simulink model "Battery_Equivalent_circuit"  (R2023b)
settings: Solver=ode23t  StartTime=0.0  StopTime=3600  MaxStep=1  RelTol=1e-3
libraries: fl_lib x11, nesl_utility x5
settings Model: Creator=prade  LastModifiedBy=prade
settings DataIOCC: SignalLoggingName=Battery_Equivalent_circuit
settings SimscapeCC: SimscapeLogType=all  SimscapeLogSimulationStatistics=on  SimscapeLogName=Battery_Equivalent_circuit

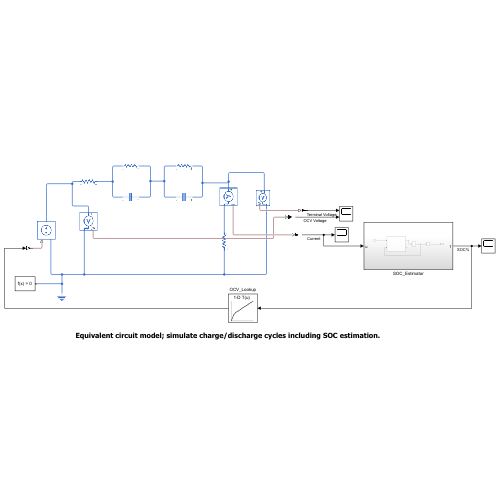
[thumbnail: Simulink's stored preview of the top-level diagram]
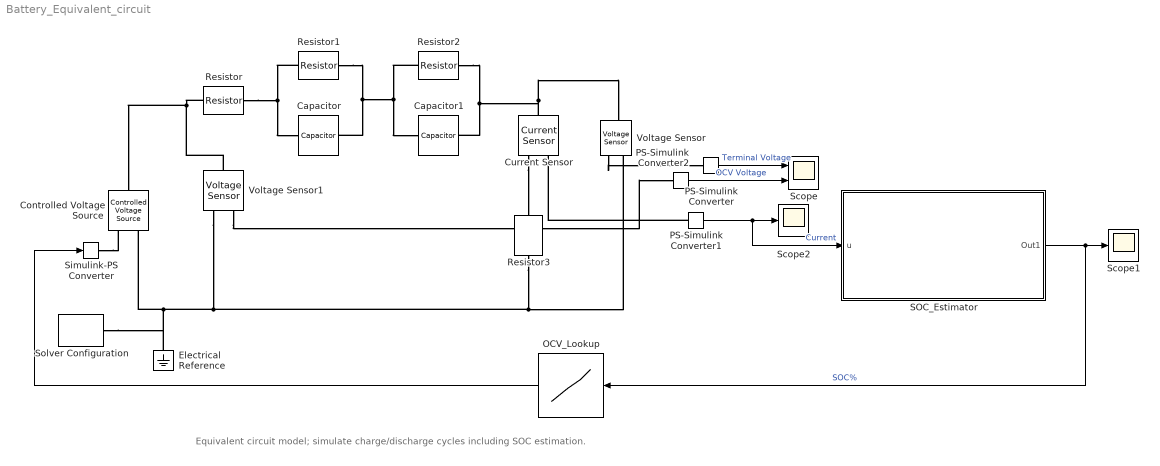
== system Battery_Equivalent_circuit ==
  note: Equivalent circuit model; simulate charge/discharge cycles including SOC estimation.
  Capacitor : fl_lib/Electrical/Electrical Elements/Capacitor  c=1000 F  r=1e-6 Ohm  g=0 1/Ohm  i_specify=off  i_priority=None  i=0 A  i_nominal_specify=off  i_nominal_unit=A  i_nominal_value=1  v_specify=off  v_priority=None  v=0 V  v_nominal_specify=off  v_nominal_unit=V  v_nominal_value=1  vc_specify=off  vc_priority=High  vc=0 V  vc_nominal_specify=off  vc_nominal_unit=V  vc_nominal_value=1
  Capacitor1 : fl_lib/Electrical/Electrical Elements/Capacitor  c=10000 F  r=1e-6 Ohm  g=0 1/Ohm  i_specify=off  i_priority=None  i=0 A  i_nominal_specify=off  i_nominal_unit=A  i_nominal_value=1  v_specify=off  v_priority=None  v=0 V  v_nominal_specify=off  v_nominal_unit=V  v_nominal_value=1  vc_specify=off  vc_priority=High  vc=0 V  vc_nominal_specify=off  vc_nominal_unit=V  vc_nominal_value=1
  Controlled Voltage Source : fl_lib/Electrical/Electrical Sources/Controlled Voltage Source
  Current Sensor : fl_lib/Electrical/Electrical Sensors/Current Sensor
  Electrical Reference : fl_lib/Electrical/Electrical Elements/Electrical Reference
  OCV_Lookup : Lookup_n-D  NumberOfTableDimensions=1  BreakpointsForDimension1=[0 10 20 30 40 50 60 70 80 90 100]  Table=[2.8 3.2 3.4 3.5 3.6 3.7 3.8 3.9 4.0 4.1 4.2]  InternalRulePriority=Speed  RndMeth=Simplest
  PS-Simulink Converter : nesl_utility/PS-Simulink Converter  PhysicalDomain=network_engine_domain  SubClassName=ps_output  LeftPortType=input  RightPortType=output  PseudoPeriodic=off  Frequencies=[]  VectorFormat=inherit  Unit=inherit  AffineConversion=off
  PS-Simulink Converter1 : nesl_utility/PS-Simulink Converter  PhysicalDomain=network_engine_domain  SubClassName=ps_output  LeftPortType=input  RightPortType=output  PseudoPeriodic=off  Frequencies=[]  VectorFormat=inherit  Unit=inherit  AffineConversion=off
  PS-Simulink Converter2 : nesl_utility/PS-Simulink Converter  PhysicalDomain=network_engine_domain  SubClassName=ps_output  LeftPortType=input  RightPortType=output  PseudoPeriodic=off  Frequencies=[]  VectorFormat=inherit  Unit=inherit  AffineConversion=off
  Resistor : fl_lib/Electrical/Electrical Elements/Resistor  R=0.05 Ohm  i_specify=off  i_priority=None  i=0 A  i_nominal_specify=off  i_nominal_unit=A  i_nominal_value=1  v_specify=off  v_priority=None  v=0 V  v_nominal_specify=off  v_nominal_unit=V  v_nominal_value=1
  Resistor1 : fl_lib/Electrical/Electrical Elements/Resistor  R=0.02 Ohm  i_specify=off  i_priority=None  i=0 A  i_nominal_specify=off  i_nominal_unit=A  i_nominal_value=1  v_specify=off  v_priority=None  v=0 V  v_nominal_specify=off  v_nominal_unit=V  v_nominal_value=1
  Resistor2 : fl_lib/Electrical/Electrical Elements/Resistor  R=0.01 Ohm  i_specify=off  i_priority=None  i=0 A  i_nominal_specify=off  i_nominal_unit=A  i_nominal_value=1  v_specify=off  v_priority=None  v=0 V  v_nominal_specify=off  v_nominal_unit=V  v_nominal_value=1
  Resistor3 : fl_lib/Electrical/Electrical Elements/Resistor  R=3.7 Ohm  i_specify=off  i_priority=None  i=0 A  i_nominal_specify=off  i_nominal_unit=A  i_nominal_value=1  v_specify=off  v_priority=None  v=0 V  v_nominal_specify=off  v_nominal_unit=V  v_nominal_value=1
  SOC_Estimator : Subsystem
  Scope : Scope  NumInputPorts=2
  Scope1 : Scope
  Scope2 : Scope
  Simulink-PS Converter : nesl_utility/Simulink-PS Converter  PhysicalDomain=network_engine_domain  SubClassName=ps_input  LeftPortType=input  RightPortType=output  PseudoPeriodic=off  Frequencies=[]  NoiseDistribution=none  NoiseParameters=[]  Unit=1  AffineConversion=off  FilteringAndDerivatives=provide  SimscapeFilterOrder=1  InputFilterTimeConstant=0.001  UdotUserProvided=0
  Solver Configuration : nesl_utility/Solver Configuration  PhysicalDomain=network_engine_domain  SubClassName=solver  LeftPortType=input  RightPortType=generic  Tones=[]  Harmonics=[]  SimulateNoise=off  Profile=off  UseLocalSampling=off  EnableSwitchedLinearOptims=on  FrequencyDomain=off  UseCCode=off  RelTol=0.001  AbsTol=0.001  MinStep=1e-09  ToWorkspace=off  RevertToSquareIcSolve=off  NumHomotopyIterations=100  PhasorMode=off  PhasorModeNumHarmonics=1  ConsistencySolver=NEWTON_XTOL_AFTER_FTOL  IndexReductionMethod=DerivativeReplacement  DoDC=off  ResidualTolerance=1e-09  ConsistencyTolSource=GLOBAL  ConsistencyAbsTol=0.001  ConsistencyRelTol=0.001  ConsistencyTolFactor=0.001  UseLocalSolver=off  LocalSolverChoice=NE_BACKWARD_EULER_ADVANCER  ResolveIndetEquations=on  FunctionEvalNumThread=1  LocalSolverSampleTime=0.001  DoFixedCost=off  MaxNonlinIter=3  MaxModeIter=2  ComputeImpulses=off  ImpulseIterations=2  LinearAlgebra=auto  LinearAlgebraNumThread=0  EquationFormulation=NE_TIME_EF  DelaysMemoryBudget=1024  AutomaticFiltering=on  FilteringTimeConstant=0.001  PartitionStorageMethod=AS_NEEDED  PartitionMemoryBudget=1024  PartitionMethod=ROBUST  MultibodyUseLocalSolver=off  MultibodyLocalSolverChoice=ODE1  MultibodyLocalSolverSampleTime=0.001
  Voltage Sensor : fl_lib/Electrical/Electrical Sensors/Voltage Sensor
  Voltage Sensor1 : fl_lib/Electrical/Electrical Sensors/Voltage Sensor
  wires:
  PS-Simulink Converter/1 -> Scope/1  "Terminal Voltage"
  SOC_Estimator/1(Out1) -> OCV_Lookup/1, Scope1/1  "SOC%"
  OCV_Lookup/1 -> Simulink-PS Converter/1
  PS-Simulink Converter2/1 -> Scope/2  "OCV Voltage"
  PS-Simulink Converter1/1 -> SOC_Estimator/1(u), Scope2/1  "Current"
  connections:
  Resistor2/LConn1 -- Current Sensor/LConn1 -- Voltage Sensor/LConn1 -- Capacitor1/LConn1
  Voltage Sensor1/LConn1 -- Resistor/RConn1 -- Controlled Voltage Source/LConn1
  Resistor3/RConn1 -- Voltage Sensor/RConn2 -- Voltage Sensor1/RConn2 -- Electrical Reference/LConn1 -- Solver Configuration/RConn1 -- Controlled Voltage Source/RConn2
  Current Sensor/RConn2 -- Resistor3/LConn1
  Voltage Sensor/RConn1 -- PS-Simulink Converter/LConn1
  PS-Simulink Converter1/LConn1 -- Current Sensor/RConn1
  Simulink-PS Converter/RConn1 -- Controlled Voltage Source/RConn1
  Voltage Sensor1/RConn1 -- PS-Simulink Converter2/LConn1
  Resistor1/RConn1 -- Capacitor/RConn1 -- Resistor/LConn1
  Resistor1/LConn1 -- Capacitor1/RConn1 -- Resistor2/RConn1 -- Capacitor/LConn1

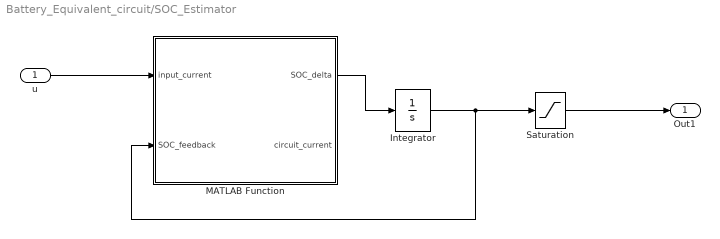
== system Battery_Equivalent_circuit/SOC_Estimator ==
  u : Inport
  Integrator : Integrator  InitialCondition=50
  MATLAB Function : MATLAB Function  TreatAsAtomicUnit=on
  Saturation : Saturate  UpperLimit=100  LowerLimit=0
  Out1 : Outport
  wires:
  u/1 -> MATLAB Function/1(input_current)
  MATLAB Function/1(SOC_delta) -> Integrator/1
  Saturation/1 -> Out1/1
  Integrator/1 -> MATLAB Function/2(SOC_feedback), Saturation/1

== matlab function Battery_Equivalent_circuit/SOC_Estimator/MATLAB Function ==
  settings: updateMethod=DISCRETE
  data: input_current input; SOC_delta output; SOC_feedback input; circuit_current output
function [SOC_delta, circuit_current] = complete_soc_with_charging(input_current, SOC_feedback)
% Complete SOC estimator that modifies both SOC calculation AND circuit current
% This ensures the battery circuit also sees the charging current

% Battery parameters
capacity_mAh = 3000;    % Adjust to your battery
timeStep = 10;           % Simulation step time

% Protection logic with hysteresis to prevent oscillation
persistent protection_active
if isempty(protection_active)
    protection_active = false;
end

% Hysteresis logic
if SOC_feedback <= 10
    protection_active = true;   % Activate charging
elseif SOC_feedback >= 99      % Turn off protection at 20%
    protection_active = false;  % Return to normal
end
% Between 10-20%, keep current state (hysteresis)

% Determine actual current for both SOC and circuit
if protection_active
    % CHARGING MODE: Reverse current direction
    circuit_current = -abs(input_current);  % Negative = charging
    eta = 0.95;  % Charging efficiency
    
    % Optional: Reduce charging current slightly for safety
    circuit_current = circuit_current * 0.8;  % 80% of discharge current
else
    % NORMAL DISCHARGE MODE
    circuit_current = input_current;  % Original current
    eta = 0.99;   % Discharge efficiency
end

% Calculate SOC change using the actual circuit current
SOC_delta = -(circuit_current * timeStep * 100 * eta) / (capacity_mAh/1000 * 3600);

end
